simulink model "UPQC_model"  (R2020b)
settings: Solver=FixedStepAuto  StartTime=0.0  StopTime=Tsim  FixedStep=Tsample  MaxStep=Tsample  RelTol=1e-3
values from neighbouring files (symbols this model uses):
  C_parallel_Series = zeros(1,4)    [Netzmodell_Ini_DL.m]    (also in workspace_Ini.mat = [1e-05 1e-05 1e-05 0])
  C_parallel_Shunt = zeros(1,4)    [Netzmodell_Ini_DL.m]    (also in workspace_Ini.mat = [1e-05 1e-05 1e-05 0])
  CC_Ki = 5    [Netzmodell_Ini_DL.m]    (also in workspace_Ini.mat)
  CC_Ki_geg = 5    [Netzmodell_Ini_DL.m]    (also in workspace_Ini.mat)
  CC_Kp = 10    [Netzmodell_Ini_DL.m]    (also in workspace_Ini.mat)
  CC_Kp_geg = 10    [Netzmodell_Ini_DL.m]    (also in workspace_Ini.mat)
  CC_OS =     [workspace_Ini.mat]
  Czk = Szenario.Czk*u    [Netzmodell_Ini_DL.m]    (also in workspace_Ini.mat = 0.003)
  fak_RVC = Szenario.fak_RVC    [Netzmodell_Ini_DL.m]    (also in workspace_Ini.mat = [1 1 1])
  fak_Uns = [1; 1; 1]    [Netzmodell_Ini_DL.m]    (also in workspace_Ini.mat = [1 1 1])
  Flicker_Schaltzeitpunkte_L1 = Schaltzeitpunkte(1,:)    [Netzmodell_Ini_DL.m]    (also in workspace_Ini.mat = 10.5)
  Flicker_Schaltzeitpunkte_L2 = Schaltzeitpunkte(2,:)    [Netzmodell_Ini_DL.m]    (also in workspace_Ini.mat = 10.5)
  Flicker_Schaltzeitpunkte_L3 = Schaltzeitpunkte(3,:)    [Netzmodell_Ini_DL.m]    (also in workspace_Ini.mat = 10.5)
  fs = [f_nom; f_nom; f_nom]    [Netzmodell_Ini_DL.m]    (also in workspace_Ini.mat = [50 50 50])
  fsw = Szenario.fsw*k    [Netzmodell_Ini_DL.m]    (also in workspace_Ini.mat = 20000)
  I_Basis_Ober_L1 = I_Basis_Ober(1)    [Netzmodell_Ini_DL.m]    (also in workspace_Ini.mat = 0)
  I_Basis_Ober_L2 = I_Basis_Ober(2)    [Netzmodell_Ini_DL.m]    (also in workspace_Ini.mat = 0)
  I_Basis_Ober_L3 = I_Basis_Ober(3)    [Netzmodell_Ini_DL.m]    (also in workspace_Ini.mat = 0)
  I_relativ_Ober_L1 = Szenario.I_relativ_Ober_L1    [Netzmodell_Ini_DL.m]    (also in workspace_Ini.mat = [0 100 0 100 100 0 100 100 0 0 0 0 ... (50 elements, 1x50)])
  I_relativ_Ober_L2 = Szenario.I_relativ_Ober_L2    [Netzmodell_Ini_DL.m]    (also in workspace_Ini.mat = [0 100 0 100 100 0 100 100 0 0 0 0 ... (50 elements, 1x50)])
  I_relativ_Ober_L3 = Szenario.I_relativ_Ober_L3    [Netzmodell_Ini_DL.m]    (also in workspace_Ini.mat = [0 100 0 100 100 0 100 100 0 0 0 0 ... (50 elements, 1x50)])
  L_Ausgang_Series = zeros(1,4)    [Netzmodell_Ini_DL.m]    (also in workspace_Ini.mat = [0.00093 0.00093 0.00093 0.00093])
  L_Ausgang_Shunt = zeros(1,4)    [Netzmodell_Ini_DL.m]    (also in workspace_Ini.mat = [0.00093 0.00093 0.00093 0.00093])
  L_Eingang_Series = zeros(1,4)    [Netzmodell_Ini_DL.m]    (also in workspace_Ini.mat = [0.00085 0.00085 0.00085 0.00085])
  L_Eingang_Shunt = zeros(1,4)    [Netzmodell_Ini_DL.m]    (also in workspace_Ini.mat = [0.00085 0.00085 0.00085 0.00085])
  Ls_in = 52.2*u/10    (= 5.22e-06)    [Netzmodell_Ini_DL.m]    (also in workspace_Ini.mat)
  Ltrans = Szenario.Ltrans*m    [Netzmodell_Ini_DL.m]    (also in workspace_Ini.mat = 0.000256)
  OS_off = 6    [Netzmodell_Ini_DL.m]    (also in workspace_Ini.mat)
  OS_on = 1    [Netzmodell_Ini_DL.m]    (also in workspace_Ini.mat)
  Phi_Ober_L1 = Phi_Ober(1)    [Netzmodell_Ini_DL.m]    (also in workspace_Ini.mat = 0)
  Phi_Ober_L2 = Phi_Ober(2)    [Netzmodell_Ini_DL.m]    (also in workspace_Ini.mat = -120)
  Phi_Ober_L3 = Phi_Ober(3)    [Netzmodell_Ini_DL.m]    (also in workspace_Ini.mat = 120)
  Phis = [0; -120; 120]    [Netzmodell_Ini_DL.m]    (also in workspace_Ini.mat = [0 -120 120])
  Pl_Flicker = Pl_Flicker*k    [Netzmodell_Ini_DL.m]    (also in workspace_Ini.mat = [5000 5000 5000])
  Pl_Grund = Szenario.Pl_Grund *k    [Netzmodell_Ini_DL.m]    (also in workspace_Ini.mat = [5 5 5])
  Pl_RVC = Pl_RVC*k    [Netzmodell_Ini_DL.m]    (also in workspace_Ini.mat = [10000 10000 10000])
  Pl_Uns = Pl_Uns*k    [Netzmodell_Ini_DL.m]    (also in workspace_Ini.mat = [25000 10 10])
  Ql_ind_Flicker = Ql_ind_Flicker*k    [Netzmodell_Ini_DL.m]    (also in workspace_Ini.mat = [0 0 0])
  Ql_ind_Grund = Szenario.Ql_ind_Grund*k    [Netzmodell_Ini_DL.m]    (also in workspace_Ini.mat = [0 0 0])
  Ql_ind_RVC = Szenario.Ql_ind_RVC*k    [Netzmodell_Ini_DL.m]    (also in workspace_Ini.mat = [0 0 0])
  Ql_ind_Uns = Ql_ind_Uns*k    [Netzmodell_Ini_DL.m]    (also in workspace_Ini.mat = [0 0 0])
  Ql_kap_Flicker = Ql_kap_Flicker*k    [Netzmodell_Ini_DL.m]    (also in workspace_Ini.mat = [0 0 0])
  Ql_kap_Grund = Szenario.Ql_kap_Grund*k    [Netzmodell_Ini_DL.m]    (also in workspace_Ini.mat = [0 0 0])
  Ql_kap_RVC = Szenario.Ql_kap_RVC*k    [Netzmodell_Ini_DL.m]    (also in workspace_Ini.mat = [0 0 0])
  Ql_kap_Uns = Ql_kap_Uns*k    [Netzmodell_Ini_DL.m]    (also in workspace_Ini.mat = [0 0 0])
  R_Ausgang_Series = zeros(1,4)    [Netzmodell_Ini_DL.m]    (also in workspace_Ini.mat = [0.1 0.1 0.1 0.1])
  R_Ausgang_Shunt = zeros(1,4)    [Netzmodell_Ini_DL.m]    (also in workspace_Ini.mat = [0.1 0.1 0.1 0.1])
  R_Eingang_Series = zeros(1,4)    [Netzmodell_Ini_DL.m]    (also in workspace_Ini.mat = [0.1 0.1 0.1 0.1])
  R_Eingang_Shunt = zeros(1,4)    [Netzmodell_Ini_DL.m]    (also in workspace_Ini.mat = [0.1 0.1 0.1 0.1])
  R_parallel_Series = zeros(1,4)    [Netzmodell_Ini_DL.m]    (also in workspace_Ini.mat = [13 13 13 0])
  R_parallel_Shunt = zeros(1,4)    [Netzmodell_Ini_DL.m]    (also in workspace_Ini.mat = [13 13 13 0])
  R_ZK_Belastung = 20    [Netzmodell_Ini_DL.m]    (also in workspace_Ini.mat)
  Rs_in = 5.2*m/10    (= 0.00052)    [Netzmodell_Ini_DL.m]    (also in workspace_Ini.mat)
  Rtrans = Szenario.Rtrans    [Netzmodell_Ini_DL.m]    (also in workspace_Ini.mat = 0.206)
  RVC_L1_on_off_Zeitpunkte = Szenario.RVC_L1_on_off_Zeitpunkte    [Netzmodell_Ini_DL.m]    (also in workspace_Ini.mat = [10.5 40 10 11 12 13 14 15])
  RVC_L2_on_off_Zeitpunkte = Szenario.RVC_L2_on_off_Zeitpunkte    [Netzmodell_Ini_DL.m]    (also in workspace_Ini.mat = [10.5 40 10 11 12 13 14 15])
  RVC_L3_on_off_Zeitpunkte = Szenario.RVC_L3_on_off_Zeitpunkte    [Netzmodell_Ini_DL.m]    (also in workspace_Ini.mat = [10.5 40 10 11 12 13 14 15])
  RVC_off = 20.5    [Netzmodell_Ini_DL.m]    (also in workspace_Ini.mat)
  RVC_on = 20    [Netzmodell_Ini_DL.m]    (also in workspace_Ini.mat)
  RVC_val = [0.8,0.8,0.8]    [Netzmodell_Ini_DL.m]    (also in workspace_Ini.mat = [0.8 0.8 0.8])
  strans = Szenario.strans    [Netzmodell_Ini_DL.m]    (also in workspace_Ini.mat = 0.25)
  t_breaker_series = tacts    [Netzmodell_Ini_DL.m]    (also in workspace_Ini.mat = 0.5)
  tact = Szenario.tact    [Netzmodell_Ini_DL.m]    (also in workspace_Ini.mat = 0.5)
  tact_OS_Regler = Szenario.tact_OS_Regler    [Netzmodell_Ini_DL.m]    (also in workspace_Ini.mat = 0.5)
  tact_QU = 10    [Netzmodell_Ini_DL.m]    (also in workspace_Ini.mat)
  tacts = Szenario.tacts    [Netzmodell_Ini_DL.m]    (also in workspace_Ini.mat = 0.5)
  Tsample = Szenario.Tsample    [Netzmodell_Ini_DL.m]    (also in workspace_Ini.mat = 5e-06)
  Uns_L1_on_off_Zeitpunkte = Szenario.Uns_L1_on_off_Zeitpunkte    [Netzmodell_Ini_DL.m]    (also in workspace_Ini.mat = [1 6 10 11 12 13 14 15])
  Uns_L2_on_off_Zeitpunkte = Szenario.Uns_L2_on_off_Zeitpunkte    [Netzmodell_Ini_DL.m]    (also in workspace_Ini.mat = [10 30 10 11 12 13 14 15])
  Uns_L3_on_off_Zeitpunkte = Szenario.Uns_L3_on_off_Zeitpunkte    [Netzmodell_Ini_DL.m]    (also in workspace_Ini.mat = [10 30 10 11 12 13 14 15])
  Us = [Us_Amp; Us_Amp; Us_Amp]    [Netzmodell_Ini_DL.m]    (also in workspace_Ini.mat = [326.598632371 326.598632371 326.598632371])
  Us_Amp = sqrt(2)*400/sqrt(3)    [Netzmodell_Ini_DL.m]    (also in workspace_Ini.mat = 326.598632371)
  VC_Ki_gegen = 30    [Netzmodell_Ini_DL.m]    (also in workspace_Ini.mat)
  VC_Ki_gegen_shunt = 15    [Netzmodell_Ini_DL.m]    (also in workspace_Ini.mat)
  VC_Ki_mit = 5    [Netzmodell_Ini_DL.m]    (also in workspace_Ini.mat)
  VC_Kp_gegen = 5    [workspace_Ini.mat]
  VC_Kp_gegen_shunt = 2    [Netzmodell_Ini_DL.m]    (also in workspace_Ini.mat)
  VC_Kp_mit = 10    [Netzmodell_Ini_DL.m]    (also in workspace_Ini.mat)
  VC_ZK_Ki = 5    [Netzmodell_Ini_DL.m]    (also in workspace_Ini.mat)
  VC_ZK_Kp = 0.5    [Netzmodell_Ini_DL.m]    (also in workspace_Ini.mat)
  Vielfache_Ober_L1 = Szenario.Vielfache_Ober_L1    [Netzmodell_Ini_DL.m]    (also in workspace_Ini.mat = [1 2 3 4 5 6 7 8 9 10 11 12 ... (50 elements, 1x50)])
  Vielfache_Ober_L2 = Szenario.Vielfache_Ober_L2    [Netzmodell_Ini_DL.m]    (also in workspace_Ini.mat = [1 2 3 4 5 6 7 8 9 10 11 12 ... (50 elements, 1x50)])
  Vielfache_Ober_L3 = Szenario.Vielfache_Ober_L3    [Netzmodell_Ini_DL.m]    (also in workspace_Ini.mat = [1 2 3 4 5 6 7 8 9 10 11 12 ... (50 elements, 1x50)])
  ZK_Belastung_off = 100    [Netzmodell_Ini_DL.m]    (also in workspace_Ini.mat)
  ZK_Belastung_on = 100    [Netzmodell_Ini_DL.m]    (also in workspace_Ini.mat)
  Zwischenkreisspannung = 700    [Netzmodell_Ini_DL.m]    (also in workspace_Ini.mat)
undefined symbols (not defined in the file or in its folder): LAusgang, RReiheL3
libraries: powerlib x221, powerlib_meascontrol x80, pid_lib x23, eeTransforms x4, eePwmGeneratorTwoLevel x2, dspstat3 x1
(part 9 of 16)

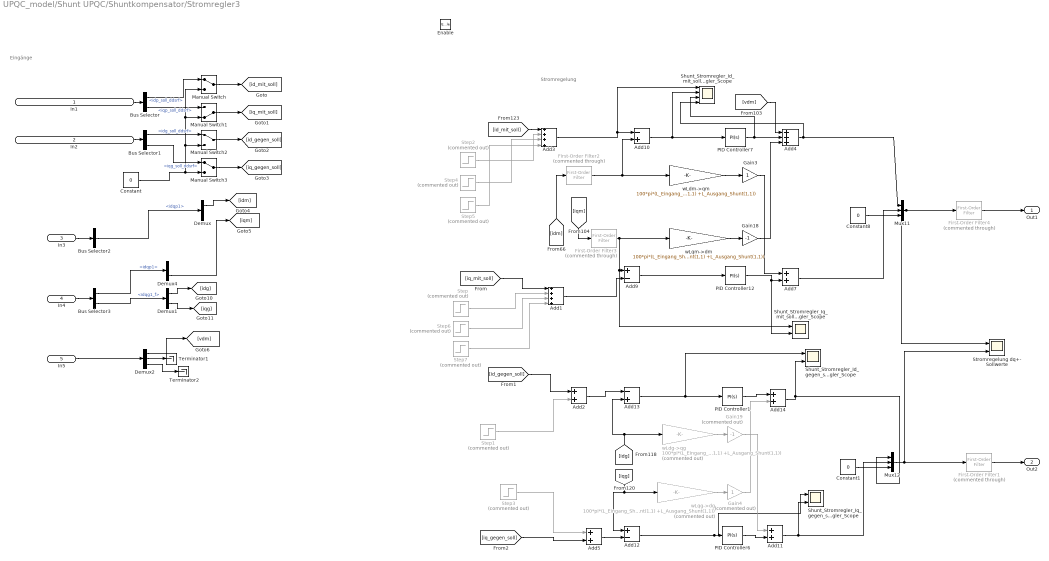
== system UPQC_model/Shunt UPQC/Shuntkompensator/Stromregler3 ==
  note: Eingänge
  note: Stromregelung
  In1 : Inport
  In2 : Inport  Port=2
  In3 : Inport  Port=3
  In4 : Inport  Port=4
  In5 : Inport  Port=5
  Enable : EnablePort
  Add1 : Sum  Inputs=++++
  Add10 : Sum  Inputs=-+
  Add{2,5,7,11,14} (5 alike) : Sum
  Add12 : Sum  Inputs=+-
  Add13 : Sum  Inputs=-+
  Add3 : Sum  Inputs=++++
  Add4 : Sum  Inputs=+++
  Add9 : Sum  Inputs=+-
  Bus Selector : BusSelector  OutputSignals=idp_soll_ddsrf,iqp_soll_ddsrf
  Bus Selector1 : BusSelector  OutputSignals=idg_soll_ddsrf,iqg_soll_ddsrf
  Bus Selector2 : BusSelector  OutputSignals=idqp1
  Bus Selector3 : BusSelector  OutputSignals=idqp1,idqg1_f
  Constant : Constant  Value=0
  Constant1 : Constant  Value=0
  Constant8 : Constant  Value=0
  Demux : Demux  Outputs=2
  Demux1 : Demux  Outputs=2
  Demux2 : Demux  Outputs=3
  Demux4 : Demux  Outputs=2
  First-Order Filter1 : powerlib_meascontrol/Filters/First-Order Filter  Commented=through  FilterType=Lowpass  Tc=1/(2*25*pi/sqrt(2))  Ts=0  Initialize=off  Vac_Init=[0, 0, 60]  Vdc_Init=0  PlotResponse=off  FreqRange="[0,  30,  1]"
  First-Order Filter2 : powerlib_meascontrol/Filters/First-Order Filter  Commented=through  FilterType=Lowpass  Tc=1/(2*5000*pi/sqrt(2))  Ts=0  Initialize=off  Vac_Init=[0, 0, 60]  Vdc_Init=0  PlotResponse=off  FreqRange="[0,  30,  1]"
  First-Order Filter3 : powerlib_meascontrol/Filters/First-Order Filter  Commented=through  FilterType=Lowpass  Tc=1/(2*5000*pi/sqrt(2))  Ts=0  Initialize=off  Vac_Init=[0, 0, 60]  Vdc_Init=0  PlotResponse=off  FreqRange="[0,  30,  1]"
  First-Order Filter4 : powerlib_meascontrol/Filters/First-Order Filter  Commented=through  FilterType=Lowpass  Tc=0.1  Ts=0  Initialize=off  Vac_Init=[0, 0, 60]  Vdc_Init=0  PlotResponse=off  FreqRange="[0,  30,  1]"
  Gain18 : Gain  Gain=-1
  Gain19 : Gain  Commented=on  Gain=-1
  Gain3 : Gain
  Gain4 : Gain  Commented=on
  Manual Switch : ManualSwitch
  Manual Switch1 : ManualSwitch  CurrentSetting=0
  Manual Switch2 : ManualSwitch
  Manual Switch3 : ManualSwitch
  Mux11 : Mux  Inputs=3
  Mux12 : Mux  Inputs=3
  PID Controller1 : pid_lib/PID Controller  Controller=PI  Form=Parallel  TimeDomain=Continuous-time  UseExternalTs=off  SampleTime=-1  IntegratorMethod=Forward Euler  FilterMethod=Forward Euler  ControllerParametersSource=internal  P=CC_Kp_geg  I=CC_Ki_geg  D=0  UseFilter=on  N=100  TunerSelectOption=Transfer Function Based (PID Tuner App)  InitialConditionSource=internal  InitialConditionForIntegrator=0  InitialConditionForFilter=0  DifferentiatorICPrevScaledInput=0  ExternalReset=none  TrackingMode=off  Kt=1  LimitOutput=off  SatLimitsSource=internal  UpperSaturationLimit=800  LowerSaturationLimit=-800  LinearizeAsGain=on  AntiWindupMode=none  Kb=1  POutMin=[]  POutMax=[]  IOutMin=[]  IOutMax=[]  DOutMin=[]  DOutMax=[]  NOutMin=[]  NOutMax=[]  SumOutMin=[]  SumOutMax=[]  SaturationOutMin=[]  SaturationOutMax=[]  PParamMin=[]  PParamMax=[]  IParamMin=[]  IParamMax=[]  DParamMin=[]  DParamMax=[]  NParamMin=[]  NParamMax=[]  KbParamMin=[]  KbParamMax=[]  KtParamMin=[]  KtParamMax=[]  KbOutMin=[]  KbOutMax=[]  KtOutMin=[]  KtOutMax=[]  IntegratorOutMin=[]  IntegratorOutMax=[]  FilterOutMin=[]  FilterOutMax=[]  SumI1OutMin=[]  SumI1OutMax=[]  SumI2OutMin=[]  SumI2OutMax=[]  SumI3OutMin=[]  SumI3OutMax=[]  SumI4OutMin=[]  SumI4OutMax=[]  SumDOutMin=[]  SumDOutMax=[]  DifferentiatorOutMin=[]  DifferentiatorOutMax=[]  FilterDiffOutCoefMin=[]  FilterDiffOutCoefMax=[]  ReciprocalOutMin=[]  ReciprocalOutMax=[]  SumDenOutMin=[]  SumDenOutMax=[]  SumNumOutMin=[]  SumNumOutMax=[]  DivideOutMin=[]  DivideOutMax=[]  UdiffTsProdOutMin=[]  UdiffTsProdOutMax=[]  NTsProdOutMin=[]  NTsProdOutMax=[]  UintegralTsProdOutMin=[]  UintegralTsProdOutMax=[]  UngainTsProdOutMin=[]  UngainTsProdOutMax=[]  IntegratorContinuousStateAttributes=''  IntegratorStateMustResolveToSignalObject=off  IntegratorRTWStateStorageClass=Auto  FilterContinuousStateAttributes=''  FilterStateMustResolveToSignalObject=off  FilterRTWStateStorageClass=Auto  ParallelPVariant=InternalParameters  IdealPVariant=Disabled  IVariant=InternalParameters  DVariant=Disabled  IntegratorVariant=Continuous  SatVariant=Disabled  AWVariant=Passthrough  PCopyVariant=Disabled  TRVariant=Disabled  FdbkBlocksVariant=Forward  IdealPFdbkVariant=Disabled  SatFdbkVariant=Disabled  DerivativeFilterVariant=Disabled  NVariant=Disabled  NCopyVariant=Disabled_SignalSpec  FilterICVariant=Disabled  IntegratorICVariant=InternalICs  ExternalResetVariant=Disabled  TRSumVariant=Passthrough  SumFdbkVariant=Disabled  SumVariant=Sum_PI  TsampFilterVariant=InternalTs  TsampNgainVariant=Passthrough  TsampIntegralVariant=Passthrough  ExternalSaturationOutDataTypeStr=Inherit: Same as second input
  PID Controller12 : pid_lib/PID Controller  Controller=PI  Form=Parallel  TimeDomain=Continuous-time  UseExternalTs=off  SampleTime=-1  IntegratorMethod=Forward Euler  FilterMethod=Forward Euler  ControllerParametersSource=internal  P=CC_Kp  I=CC_Ki  D=0  UseFilter=on  N=100  TunerSelectOption=Transfer Function Based (PID Tuner App)  InitialConditionSource=internal  InitialConditionForIntegrator=0  InitialConditionForFilter=0  DifferentiatorICPrevScaledInput=0  ExternalReset=none  TrackingMode=off  Kt=1  LimitOutput=off  SatLimitsSource=internal  UpperSaturationLimit=800  LowerSaturationLimit=-800  LinearizeAsGain=on  AntiWindupMode=none  Kb=1  POutMin=[]  POutMax=[]  IOutMin=[]  IOutMax=[]  DOutMin=[]  DOutMax=[]  NOutMin=[]  NOutMax=[]  SumOutMin=[]  SumOutMax=[]  SaturationOutMin=[]  SaturationOutMax=[]  PParamMin=[]  PParamMax=[]  IParamMin=[]  IParamMax=[]  DParamMin=[]  DParamMax=[]  NParamMin=[]  NParamMax=[]  KbParamMin=[]  KbParamMax=[]  KtParamMin=[]  KtParamMax=[]  KbOutMin=[]  KbOutMax=[]  KtOutMin=[]  KtOutMax=[]  IntegratorOutMin=[]  IntegratorOutMax=[]  FilterOutMin=[]  FilterOutMax=[]  SumI1OutMin=[]  SumI1OutMax=[]  SumI2OutMin=[]  SumI2OutMax=[]  SumI3OutMin=[]  SumI3OutMax=[]  SumI4OutMin=[]  SumI4OutMax=[]  SumDOutMin=[]  SumDOutMax=[]  DifferentiatorOutMin=[]  DifferentiatorOutMax=[]  FilterDiffOutCoefMin=[]  FilterDiffOutCoefMax=[]  ReciprocalOutMin=[]  ReciprocalOutMax=[]  SumDenOutMin=[]  SumDenOutMax=[]  SumNumOutMin=[]  SumNumOutMax=[]  DivideOutMin=[]  DivideOutMax=[]  UdiffTsProdOutMin=[]  UdiffTsProdOutMax=[]  NTsProdOutMin=[]  NTsProdOutMax=[]  UintegralTsProdOutMin=[]  UintegralTsProdOutMax=[]  UngainTsProdOutMin=[]  UngainTsProdOutMax=[]  IntegratorContinuousStateAttributes=''  IntegratorStateMustResolveToSignalObject=off  IntegratorRTWStateStorageClass=Auto  FilterContinuousStateAttributes=''  FilterStateMustResolveToSignalObject=off  FilterRTWStateStorageClass=Auto  ParallelPVariant=InternalParameters  IdealPVariant=Disabled  IVariant=InternalParameters  DVariant=Disabled  IntegratorVariant=Continuous  SatVariant=Disabled  AWVariant=Passthrough  PCopyVariant=Disabled  TRVariant=Disabled  FdbkBlocksVariant=Forward  IdealPFdbkVariant=Disabled  SatFdbkVariant=Disabled  DerivativeFilterVariant=Disabled  NVariant=Disabled  NCopyVariant=Disabled_SignalSpec  FilterICVariant=Disabled  IntegratorICVariant=InternalICs  ExternalResetVariant=Disabled  TRSumVariant=Passthrough  SumFdbkVariant=Disabled  SumVariant=Sum_PI  TsampFilterVariant=InternalTs  TsampNgainVariant=Passthrough  TsampIntegralVariant=Passthrough  ExternalSaturationOutDataTypeStr=Inherit: Same as second input
  PID Controller6 : pid_lib/PID Controller  Controller=PI  Form=Parallel  TimeDomain=Continuous-time  UseExternalTs=off  SampleTime=-1  IntegratorMethod=Forward Euler  FilterMethod=Forward Euler  ControllerParametersSource=internal  P=CC_Kp_geg  I=CC_Ki_geg  D=0  UseFilter=on  N=100  TunerSelectOption=Transfer Function Based (PID Tuner App)  InitialConditionSource=internal  InitialConditionForIntegrator=0  InitialConditionForFilter=0  DifferentiatorICPrevScaledInput=0  ExternalReset=none  TrackingMode=off  Kt=1  LimitOutput=off  SatLimitsSource=internal  UpperSaturationLimit=800  LowerSaturationLimit=-800  LinearizeAsGain=on  AntiWindupMode=none  Kb=1  POutMin=[]  POutMax=[]  IOutMin=[]  IOutMax=[]  DOutMin=[]  DOutMax=[]  NOutMin=[]  NOutMax=[]  SumOutMin=[]  SumOutMax=[]  SaturationOutMin=[]  SaturationOutMax=[]  PParamMin=[]  PParamMax=[]  IParamMin=[]  IParamMax=[]  DParamMin=[]  DParamMax=[]  NParamMin=[]  NParamMax=[]  KbParamMin=[]  KbParamMax=[]  KtParamMin=[]  KtParamMax=[]  KbOutMin=[]  KbOutMax=[]  KtOutMin=[]  KtOutMax=[]  IntegratorOutMin=[]  IntegratorOutMax=[]  FilterOutMin=[]  FilterOutMax=[]  SumI1OutMin=[]  SumI1OutMax=[]  SumI2OutMin=[]  SumI2OutMax=[]  SumI3OutMin=[]  SumI3OutMax=[]  SumI4OutMin=[]  SumI4OutMax=[]  SumDOutMin=[]  SumDOutMax=[]  DifferentiatorOutMin=[]  DifferentiatorOutMax=[]  FilterDiffOutCoefMin=[]  FilterDiffOutCoefMax=[]  ReciprocalOutMin=[]  ReciprocalOutMax=[]  SumDenOutMin=[]  SumDenOutMax=[]  SumNumOutMin=[]  SumNumOutMax=[]  DivideOutMin=[]  DivideOutMax=[]  UdiffTsProdOutMin=[]  UdiffTsProdOutMax=[]  NTsProdOutMin=[]  NTsProdOutMax=[]  UintegralTsProdOutMin=[]  UintegralTsProdOutMax=[]  UngainTsProdOutMin=[]  UngainTsProdOutMax=[]  IntegratorContinuousStateAttributes=''  IntegratorStateMustResolveToSignalObject=off  IntegratorRTWStateStorageClass=Auto  FilterContinuousStateAttributes=''  FilterStateMustResolveToSignalObject=off  FilterRTWStateStorageClass=Auto  ParallelPVariant=InternalParameters  IdealPVariant=Disabled  IVariant=InternalParameters  DVariant=Disabled  IntegratorVariant=Continuous  SatVariant=Disabled  AWVariant=Passthrough  PCopyVariant=Disabled  TRVariant=Disabled  FdbkBlocksVariant=Forward  IdealPFdbkVariant=Disabled  SatFdbkVariant=Disabled  DerivativeFilterVariant=Disabled  NVariant=Disabled  NCopyVariant=Disabled_SignalSpec  FilterICVariant=Disabled  IntegratorICVariant=InternalICs  ExternalResetVariant=Disabled  TRSumVariant=Passthrough  SumFdbkVariant=Disabled  SumVariant=Sum_PI  TsampFilterVariant=InternalTs  TsampNgainVariant=Passthrough  TsampIntegralVariant=Passthrough  ExternalSaturationOutDataTypeStr=Inherit: Same as second input
  PID Controller7 : pid_lib/PID Controller  Controller=PI  Form=Parallel  TimeDomain=Continuous-time  UseExternalTs=off  SampleTime=-1  IntegratorMethod=Forward Euler  FilterMethod=Forward Euler  ControllerParametersSource=internal  P=CC_Kp  I=CC_Ki  D=0  UseFilter=on  N=100  TunerSelectOption=Transfer Function Based (PID Tuner App)  InitialConditionSource=internal  InitialConditionForIntegrator=0  InitialConditionForFilter=0  DifferentiatorICPrevScaledInput=0  ExternalReset=none  TrackingMode=off  Kt=1  LimitOutput=off  SatLimitsSource=internal  UpperSaturationLimit=800  LowerSaturationLimit=-800  LinearizeAsGain=on  AntiWindupMode=none  Kb=1  POutMin=[]  POutMax=[]  IOutMin=[]  IOutMax=[]  DOutMin=[]  DOutMax=[]  NOutMin=[]  NOutMax=[]  SumOutMin=[]  SumOutMax=[]  SaturationOutMin=[]  SaturationOutMax=[]  PParamMin=[]  PParamMax=[]  IParamMin=[]  IParamMax=[]  DParamMin=[]  DParamMax=[]  NParamMin=[]  NParamMax=[]  KbParamMin=[]  KbParamMax=[]  KtParamMin=[]  KtParamMax=[]  KbOutMin=[]  KbOutMax=[]  KtOutMin=[]  KtOutMax=[]  IntegratorOutMin=[]  IntegratorOutMax=[]  FilterOutMin=[]  FilterOutMax=[]  SumI1OutMin=[]  SumI1OutMax=[]  SumI2OutMin=[]  SumI2OutMax=[]  SumI3OutMin=[]  SumI3OutMax=[]  SumI4OutMin=[]  SumI4OutMax=[]  SumDOutMin=[]  SumDOutMax=[]  DifferentiatorOutMin=[]  DifferentiatorOutMax=[]  FilterDiffOutCoefMin=[]  FilterDiffOutCoefMax=[]  ReciprocalOutMin=[]  ReciprocalOutMax=[]  SumDenOutMin=[]  SumDenOutMax=[]  SumNumOutMin=[]  SumNumOutMax=[]  DivideOutMin=[]  DivideOutMax=[]  UdiffTsProdOutMin=[]  UdiffTsProdOutMax=[]  NTsProdOutMin=[]  NTsProdOutMax=[]  UintegralTsProdOutMin=[]  UintegralTsProdOutMax=[]  UngainTsProdOutMin=[]  UngainTsProdOutMax=[]  IntegratorContinuousStateAttributes=''  IntegratorStateMustResolveToSignalObject=off  IntegratorRTWStateStorageClass=Auto  FilterContinuousStateAttributes=''  FilterStateMustResolveToSignalObject=off  FilterRTWStateStorageClass=Auto  ParallelPVariant=InternalParameters  IdealPVariant=Disabled  IVariant=InternalParameters  DVariant=Disabled  IntegratorVariant=Continuous  SatVariant=Disabled  AWVariant=Passthrough  PCopyVariant=Disabled  TRVariant=Disabled  FdbkBlocksVariant=Forward  IdealPFdbkVariant=Disabled  SatFdbkVariant=Disabled  DerivativeFilterVariant=Disabled  NVariant=Disabled  NCopyVariant=Disabled_SignalSpec  FilterICVariant=Disabled  IntegratorICVariant=InternalICs  ExternalResetVariant=Disabled  TRSumVariant=Passthrough  SumFdbkVariant=Disabled  SumVariant=Sum_PI  TsampFilterVariant=InternalTs  TsampNgainVariant=Passthrough  TsampIntegralVariant=Passthrough  ExternalSaturationOutDataTypeStr=Inherit: Same as second input
  Shunt_Stromregler_Id_gegen_soll_vor_nach_PIRegler_Scope : Scope  NumInputPorts=2
  Shunt_Stromregler_Id_mit_soll_vor_nach_PIRegler_Scope : Scope  NumInputPorts=4
  Shunt_Stromregler_Iq_gegen_soll_vor_nach_PIRegler_Scope : Scope  NumInputPorts=2
  Shunt_Stromregler_Iq_mit_soll_vor_nach_PIRegler_Scope : Scope  NumInputPorts=2
  Step : Step  Commented=on  Time=0.5  After=20  SampleTime=0
  Step1 : Step  Commented=on  Time=0  After=0  SampleTime=0
  Step2 : Step  Commented=on  After=20  SampleTime=0
  Step3 : Step  Commented=on  Time=0  After=0  SampleTime=0
  Step4 : Step  Commented=on  Time=1.3  After=-40  SampleTime=0
  Step5 : Step  Commented=on  Time=1.6  After=20  SampleTime=0
  Step6 : Step  Commented=on  After=-40  SampleTime=0
  Step7 : Step  Commented=on  Time=1.5  After=20  SampleTime=0
  Stromregelung dq+- Sollwerte : Scope  NumInputPorts=2
  Terminator1 : Terminator
  Terminator2 : Terminator
  wLdg->qg : Gain  Commented=on  Gain=100*pi*(L_Eingang_Shunt(1,1) +L_Ausgang_Shunt(1,1))
  wLdm->qm : Gain  Gain=100*pi*(L_Eingang_Shunt(1,1) +L_Ausgang_Shunt(1,1))
  wLqg->dg : Gain  Commented=on  Gain=100*pi*(L_Eingang_Shunt(1,1) +L_Ausgang_Shunt(1,1))
  wLqm->dm : Gain  Gain=100*pi*(L_Eingang_Shunt(1,1) +L_Ausgang_Shunt(1,1))
  Out1 : Outport
  Out2 : Outport  Port=2
  wires:
  Add9/1 -> PID Controller12/1
  Add10/1 -> Shunt_Stromregler_Id_mit_soll_vor_nach_PIRegler_Scope/2, PID Controller7/1
  [iqm] -> First-Order Filter3/1
  Add12/1 -> Shunt_Stromregler_Iq_gegen_soll_vor_nach_PIRegler_Scope/1, PID Controller6/1
  [idg] -> Add13/2, wLdg->qg/1
  Add13/1 -> Shunt_Stromregler_Id_gegen_soll_vor_nach_PIRegler_Scope/1, PID Controller1/1
  wLdm->qm/1 -> Gain3/1
  [idm] -> First-Order Filter2/1
  Mux12/1 -> Stromregelung dq+- Sollwerte/2, First-Order Filter1/1
  Constant8/1 -> Mux11/3
  wLqm->dm/1 -> Gain18/1
  Gain18/1 -> Add4/3
  Gain19/1 -> Add11/1
  PID Controller12/1 -> Shunt_Stromregler_Iq_mit_soll_vor_nach_PIRegler_Scope/2, Add7/2
  PID Controller6/1 -> Add11/2
  PID Controller7/1 -> Shunt_Stromregler_Id_mit_soll_vor_nach_PIRegler_Scope/3, Add4/2
  wLdg->qg/1 -> Gain19/1
  PID Controller1/1 -> Add14/1
  [vdm] -> Add4/1
  [iqg] -> Add12/1, wLqg->dg/1
  wLqg->dg/1 -> Gain4/1
  In1/1 -> Bus Selector/1
  In2/1 -> Bus Selector1/1
  In3/1 -> Bus Selector2/1
  In5/1 -> Demux2/1
  Bus Selector/1 -> Manual Switch/1  "<idp_soll_ddsrf>"
  Bus Selector/2 -> Manual Switch1/1  "<iqp_soll_ddsrf>"
  Bus Selector1/1 -> Manual Switch2/1  "<idg_soll_ddsrf>"
  Bus Selector1/2 -> Manual Switch3/1  "<iqg_soll_ddsrf>"
  Demux2/3 -> Terminator2/1
  Demux2/1 -> [vdm]
  [id_gegen_soll] -> Add2/1
  Step/1 -> Add1/2
  Add2/1 -> Add13/1
  Step1/1 -> Add2/2
  Mux11/1 -> First-Order Filter4/1, Stromregelung dq+- Sollwerte/1
  Add7/1 -> Mux11/2
  [iq_mit_soll] -> Add1/1
  Manual Switch/1 -> [id_mit_soll]
  Manual Switch1/1 -> [iq_mit_soll]
  Manual Switch2/1 -> [id_gegen_soll]
  Manual Switch3/1 -> [iq_gegen_soll]
  Constant/1 -> Manual Switch/2, Manual Switch1/2, Manual Switch2/2, Manual Switch3/2
  Constant1/1 -> Mux12/3
  Add3/1 -> Shunt_Stromregler_Id_mit_soll_vor_nach_PIRegler_Scope/1, Add10/1
  Demux/1 -> [idm]
  Demux1/1 -> [idg]
  Demux1/2 -> [iqg]
  Gain3/1 -> Add7/1
  Gain4/1 -> Add14/2
  [id_mit_soll] -> Add3/1
  Step2/1 -> Add3/2
  Add5/1 -> Add12/2
  [iq_gegen_soll] -> Add5/2
  Step3/1 -> Add5/1
  First-Order Filter1/1 -> Out2/1
  Bus Selector2/1 -> Demux/1  "<idqp1>"
  Step4/1 -> Add3/3
  Step5/1 -> Add3/4
  Step6/1 -> Add1/3
  Step7/1 -> Add1/4
  Add1/1 -> Add9/2
  Add14/1 -> Mux12/1, Shunt_Stromregler_Id_gegen_soll_vor_nach_PIRegler_Scope/2
  Add11/1 -> Mux12/2, Shunt_Stromregler_Iq_gegen_soll_vor_nach_PIRegler_Scope/2
  First-Order Filter2/1 -> wLdm->qm/1, Add10/2
  First-Order Filter3/1 -> wLqm->dm/1, Add9/1, Shunt_Stromregler_Iq_mit_soll_vor_nach_PIRegler_Scope/1
  In4/1 -> Bus Selector3/1
  Bus Selector3/2 -> Demux1/1  "<idqg1_f>"
  Bus Selector3/1 -> Demux4/1  "<idqp1>"
  Demux4/2 -> [iqm]
  First-Order Filter4/1 -> Out1/1
  Add4/1 -> Mux11/1, Shunt_Stromregler_Id_mit_soll_vor_nach_PIRegler_Scope/4
  Demux2/2 -> Terminator1/1

== system UPQC_model/Shunt UPQC/Shuntkompensator/Subsystem1 ==
  upos : Inport
  phiPLL : Inport  Port=2
  uneg : Inport  Port=3
  100Hz : Inport  Port=4
  200Hz : Inport  Port=5
  250Hz : Inport  Port=6
  350Hz : Inport  Port=7
  400Hz : Inport  Port=8
  950Hz : Inport  Port=9
  Add1 : Sum  Inputs=++++++++
  Add2 : Sum  Inputs=++++++++
  Add3 : Sum
  Add4 : Sum  Commented=on
  Alpha-Beta-Zero to abc{,1..3} (4 alike) : powerlib_meascontrol/Transformations/Alpha-Beta-Zero to abc
      settings: SourceProductBaseCode=PS
  Constant : Constant  Value=0
  Demux : Demux  Outputs=3
  Demux{1,3..7} (6 alike) : Demux  Outputs=2
  Demux2 : Demux  Outputs=3
  Gain1 : Gain  Gain=-1
  Gain2 : Gain  Gain=-4
  Gain3 : Gain  Gain=5
  Gain4 : Gain  Gain=2
  Gain5 : Gain  Gain=-7
  Gain6 : Gain  Gain=8
  Gain7 : Gain  Gain=-19
  Mux{1..4} (4 alike) : Mux  Inputs=3
  SP_mitgegenalphabeta_Scope : Scope  NumInputPorts=4
  Tdq+1_1 : Subsystem
  Tdq+1_2 : Subsystem
  Tdq+1_3 : Subsystem
  Tdq+1_4 : Subsystem
  Tdq+1_5 : Subsystem
  Tdq+1_6 : Subsystem
  Tdq+2 : Subsystem
  Tdq+3 : Subsystem
  Terminator : Terminator
  Uab0mitUab0gegen_addiert_Scope : Scope
  Uabc_Signale_Scope : Scope  NumInputPorts=3
  sp : Outport
  wires:
  Mux2/1 -> Alpha-Beta-Zero to abc/1
  Add2/1 -> Mux2/2
  Add1/1 -> Mux2/1
  upos/1 -> Tdq+2/1(upos)
  uneg/1 -> Tdq+3/1(uneg)
  Demux2/3 -> Add3/2
  Demux/3 -> Add3/1
  Add3/1 -> Terminator/1
  Tdq+2/1(Out1) -> Add4/1, Demux/1
  Tdq+3/1(Out1) -> Add4/2, Demux2/1
  Demux/1 -> SP_mitgegenalphabeta_Scope/1, Mux4/1, Add1/1
  Demux2/1 -> SP_mitgegenalphabeta_Scope/2, Add1/2
  Demux2/2 -> SP_mitgegenalphabeta_Scope/4, Add2/2
  Demux/2 -> Mux4/2, SP_mitgegenalphabeta_Scope/3, Add2/1
  phiPLL/1 -> Gain4/1, Gain7/1, Gain6/1, Gain5/1, Gain3/1, Gain2/1, Tdq+3/2(phiPLL), Gain1/1
  Add4/1 -> Uab0mitUab0gegen_addiert_Scope/1
  Gain1/1 -> Tdq+2/2(phiPLL)
  Alpha-Beta-Zero to abc/1 -> sp/1
  200Hz/1 -> Tdq+1_1/1(In1)
  Gain2/1 -> Tdq+1_1/2(In2)
  Gain3/1 -> Tdq+1_2/2(In2)
  Tdq+1_1/1(Out1) -> Demux1/1  "iab4"
  Tdq+1_2/1(Out1) -> Demux3/1  "idqp1"
  Demux1/1 -> Add1/3, Mux1/1
  Demux3/1 -> Add1/4, Mux3/1
  Demux1/2 -> Add2/3, Mux1/2
  Demux3/2 -> Add2/4, Mux3/2
  250Hz/1 -> Tdq+1_2/1(In1)
  Mux1/1 -> Alpha-Beta-Zero to abc1/1
  Mux3/1 -> Alpha-Beta-Zero to abc2/1
  Constant/1 -> Mux1/3, Mux3/3, Mux4/3, Mux2/3
  Alpha-Beta-Zero to abc1/1 -> Uabc_Signale_Scope/2
  Alpha-Beta-Zero to abc2/1 -> Uabc_Signale_Scope/3
  Mux4/1 -> Alpha-Beta-Zero to abc3/1
  Alpha-Beta-Zero to abc3/1 -> Uabc_Signale_Scope/1
  100Hz/1 -> Tdq+1_3/1(100Hz)
  Gain4/1 -> Tdq+1_3/2(In2)
  Tdq+1_3/1(Out1) -> Demux4/1  "idqp1"
  350Hz/1 -> Tdq+1_4/1(350Hz)
  400Hz/1 -> Tdq+1_5/1(350Hz)
  950Hz/1 -> Tdq+1_6/1(350Hz)
  Tdq+1_4/1(Out1) -> Demux5/1  "idqp1"
  Tdq+1_5/1(Out1) -> Demux6/1  "idqp1"
  Tdq+1_6/1(Out1) -> Demux7/1  "idqp1"
  Gain5/1 -> Tdq+1_4/2(In2)
  Gain6/1 -> Tdq+1_5/2(In2)
  Gain7/1 -> Tdq+1_6/2(In2)
  Demux4/1 -> Add1/5
  Demux5/1 -> Add1/6
  Demux6/1 -> Add1/7
  Demux7/1 -> Add1/8
  Demux4/2 -> Add2/5
  Demux5/2 -> Add2/6
  Demux6/2 -> Add2/7
  Demux7/2 -> Add2/8

== system UPQC_model/Shunt UPQC/Shuntkompensator/Subsystem4 ==
  dVdc : Inport
  Constant1 : Constant  Value=0
  Step1 : Step  Time=tact  SampleTime=0
  Switch : Switch  Criteria=u2 > Threshold
  Gatesignale_(6) : Outport
  wires:
  Switch/1 -> Gatesignale_(6)/1
  dVdc/1 -> Switch/1
  Constant1/1 -> Switch/3
  Step1/1 -> Switch/2

== system UPQC_model/Shunt UPQC/Shuntkompensator/Subsystem7 ==
  dVdc : Inport
  Constant1 : Constant  Value=0
  Step1 : Step  Time=tact  SampleTime=0
  Switch : Switch  Criteria=u2 > Threshold
  Gatesignale_(6) : Outport
  wires:
  Step1/1 -> Switch/2
  Constant1/1 -> Switch/3
  dVdc/1 -> Switch/1
  Switch/1 -> Gatesignale_(6)/1
